simulink model "sldemo_tank"  (R2019b)
settings: Solver=ode1  StartTime=0.0  StopTime=170  FixedStep=.5  RelTol=1e-3  AbsTol=1e-6
PreLoadFcn:
  | sldemo_tankgui
StartFcn:
  | sldemo_tankgui start
StopFcn:
  | sldemo_tankgui stop
undefined symbols (not defined in the file): area, hilim, inflow, lolim, outflow, sigbuilder_block
CloseFcn:
  | sldemo_tankgui done
Description:
  | Tank Fill and Empty with Animation
  | 
  | This example shows how to model the dynamics of liquid in a tank. The
  | associated animation provides a graphical display of the tank as it empties and
  | refills, based on user-defined tank parameters. The tank empties at the start
  | of the simulation and again part way through the simulation. When the simulation
  | is stopped, a plot is generated showing the liquid height and the states of the
  | two valves.
settings Model: ExtModeTrigMode=oneshot  ExtModeArmWhenConnect=off  ExtModeAutoUpdateStatusClock=off  Creator=The MathWorks, Inc.  LastModifiedBy=The MathWorks, Inc.
settings SolverCC: AutoScaleAbsTol=off
settings DataIOCC: SaveFormat=Array  ReturnWorkspaceOutputs=off  SignalLoggingName=sigsOut
settings OptimizationCC: InitFltsAndDblsToZero=on  LifeSpan=inf  BufferReusableBoundary=off
settings DebuggingCC: SaveWithParameterizedLinksMsg=none  UnderspecifiedInitializationDetection=Classic  MergeDetectMultiDrivingBlocksExec=none  SignalResolutionControl=TryResolveAllWithWarning  MultiTaskDSMMsg=warning  MultiTaskCondExecSysMsg=none  IntegerOverflowMsg=none  FcnCallInpInsideContextMsg=warning  BusObjectLabelMismatch=none  StateNameClashWarn=warning  SFUnexpectedBacktrackingDiag=warning  SFNoUnconditionalDefaultTransitionDiag=warning  SFExecutionAtInitializationDiag=none  IntegerSaturationMsg=none  ArithmeticOperatorsInVariantConditions=warning
settings HardwareCC: ProdBitPerPointer=32  ProdBitPerSizeT=32  ProdBitPerPtrDiffT=32  ProdLargestAtomicFloat=None  ProdIntDivRoundTo=Undefined  ProdEndianess=Unspecified  ProdWordSize=32  ProdHWDeviceType=32-bit Generic  TargetUnknown=on
settings ModelReferenceCC: PropagateSignalLabelsOutOfModel=off
settings SFSimCC: SimUseLocalCustomCode=off  CustomCodeUndefinedFunction=UseInterfaceOnly
settings RTWCC: Description=Generic Real-Time Target  RTWUseLocalCustomCode=off
settings CodeAppCC: StateflowObjectComments=on
settings GRTTargetCC: TargetFcnLib=ansi_tfl_tmw.mat  TargetLangStandard=C89/C90 (ANSI)  GeneratePreprocessorConditionals=Disable all  CombineOutputUpdateFcns=off  GRTInterface=on
settings ConfigComp: CovMetricSettings=dw  CovHtmlReporting=on  CovSaveCumulativeToWorkspaceVar=on  CovSaveSingleToWorkspaceVar=on  CovExternalEMLEnable=off

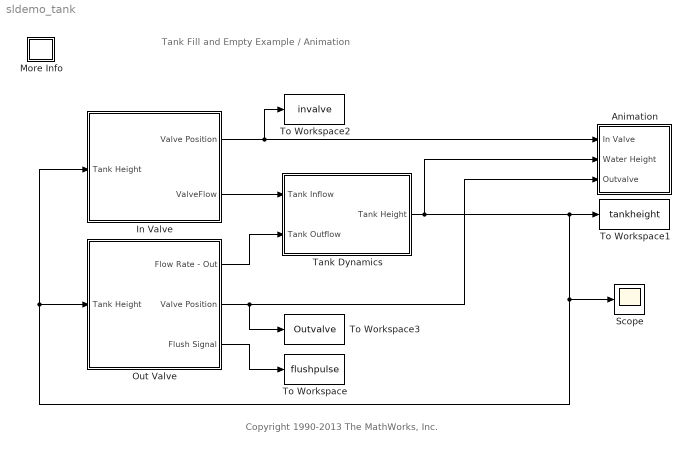
== system sldemo_tank ==
  note: Tank Fill and Empty Example / Animation
  note: Copyright 1990-2013 The MathWorks, Inc.
  Animation : Subsystem
      mask Display: disp('Animation\nControl')
  In Valve : Subsystem  mask{hilim=hilim, inflow=inflow}
      mask prompts: hilim "Shut Off Height"; inflow "Flow Rate"
  More Info : Subsystem
      settings: OpenFcn=showExample('simulink_general/sldemo_tankExample')
      mask Display: disp('?')
  Out Valve : Subsystem
  Scope : Scope
  Tank Dynamics : Subsystem
  To Workspace : ToWorkspace  VariableName=flushpulse  SampleTime=-1
  To Workspace1 : ToWorkspace  VariableName=tankheight  SampleTime=-1
  To Workspace2 : ToWorkspace  VariableName=invalve  SampleTime=-1
  To Workspace3 : ToWorkspace  VariableName=Outvalve  SampleTime=-1
  wires:
  Out Valve/2(Valve Position) -> Animation/3(Outvalve), To Workspace3/1
  In Valve/1(Valve Position) -> Animation/1(In Valve), To Workspace2/1
  Tank Dynamics/1(Tank Height) -> Animation/2(Water Height), Scope/1, In Valve/1(Tank Height), Out Valve/1(Tank Height), To Workspace1/1
  In Valve/2(ValveFlow) -> Tank Dynamics/1(Tank Inflow)
  Out Valve/1(Flow Rate - Out) -> Tank Dynamics/2(Tank Outflow)
  Out Valve/3(Flush Signal) -> To Workspace/1

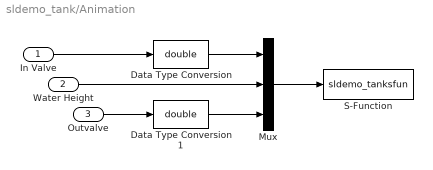
== system sldemo_tank/Animation ==
  In Valve : Inport
  Water Height : Inport  Port=2
  Outvalve : Inport  Port=3
  Data Type Conversion : DataTypeConversion  OutDataTypeStr=double  SaturateOnIntegerOverflow=on  RndMeth=Zero
  Data Type Conversion1 : DataTypeConversion  OutDataTypeStr=double  SaturateOnIntegerOverflow=on  RndMeth=Zero
  Mux : Mux  Inputs=3
  S-Function : S-Function  FunctionName=sldemo_tanksfun  Parameters=inflow,outflow,lolim,hilim,area  SFunctionDeploymentMode=off  EnableBusSupport=off
  wires:
  Outvalve/1 -> Data Type Conversion1/1
  Water Height/1 -> Mux/2
  Mux/1 -> S-Function/1
  In Valve/1 -> Data Type Conversion/1
  Data Type Conversion1/1 -> Mux/3
  Data Type Conversion/1 -> Mux/1

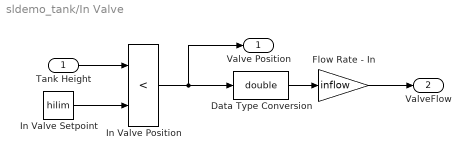
== system sldemo_tank/In Valve ==
  Tank Height : Inport
  Data Type Conversion : DataTypeConversion  OutDataTypeStr=double  SaturateOnIntegerOverflow=on  RndMeth=Zero
  Flow Rate - In : Gain  Gain=inflow  OutDataTypeStr=Inherit: Inherit via back propagation  SaturateOnIntegerOverflow=on  ParamDataTypeStr=Inherit: Same as input
  In Valve Position : RelationalOperator  Operator=<  RndMeth=Nearest  InputSameDT=on
  In Valve Setpoint : Constant  Value=hilim
  Valve Position : Outport  InitialOutput=0  VectorParamsAs1DForOutWhenUnconnected=off
  ValveFlow : Outport  Port=2  InitialOutput=0  VectorParamsAs1DForOutWhenUnconnected=off
  wires:
  Flow Rate - In/1 -> ValveFlow/1
  In Valve Position/1 -> Valve Position/1, Data Type Conversion/1
  Tank Height/1 -> In Valve Position/1
  In Valve Setpoint/1 -> In Valve Position/2
  Data Type Conversion/1 -> Flow Rate - In/1

== system sldemo_tank/More Info ==

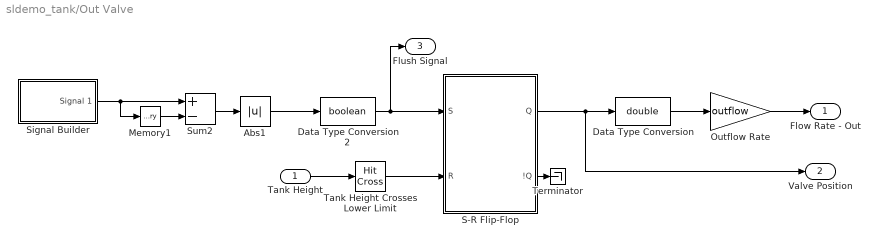
== system sldemo_tank/Out Valve ==
  Tank Height : Inport
  Abs1 : Abs  SaturateOnIntegerOverflow=on
  Data Type Conversion2 : DataTypeConversion  OutDataTypeStr=boolean  SaturateOnIntegerOverflow=on  RndMeth=Zero
  Data Type Conversion : DataTypeConversion  OutDataTypeStr=double  SaturateOnIntegerOverflow=on  RndMeth=Zero
  Memory1 : Memory
  Outflow Rate : Gain  Gain=outflow  SaturateOnIntegerOverflow=on  OutDataTypeStr=Inherit: Same as input  ParamDataTypeStr=Inherit: Same as input
  S-R Flip-Flop : Subsystem  mask(S-R Flip-Flop){}
  Signal Builder : Subsystem  Tag=STV Subsys  LoadFcn=sigbuilder_block('load');  StartFcn=sigbuilder_block('start');  StopFcn=sigbuilder_block('stop');  ClipboardFcn=sigbuilder_block('clipboard');  mask(Sigbuilder block){tuvar=[0:10]}
      mask help: Sigbuilder GUI
      mask init:
      | if ~strcmp(get_param(bdroot(gcb),'SimulationStatus'),'stopped') tuvar = sigbuilder_block('maskInit'); end
      settings: CopyFcn=sigbuilder_block('copy');  DeleteFcn=sigbuilder_block('delete');  ModelCloseFcn=sigbuilder_block('modelClose');  PreSaveFcn=sigbuilder_block('preSave');  PauseFcn=sigbuilder_block('pause')  ContinueFcn=sigbuilder_block('continue')  NameChangeFcn=sigbuilder_block('namechange');  OpenFcn=sigbuilder_block('open',[87.75 166.5 618.75 375 ]);  CloseFcn=sigbuilder_block('close');
      mask Display: plot(0, 0, 100, 100,[2, 2, 32, 32, 2], [68, 8, 8, 68, 68],[32, 2], [38, 38], [32, 19, 2],[53, 60, 44], [32, 17, 17, 2],[16, 16, 31, 31]);txt = getActiveGroup(gcbh);text(2, 100, txt,'verticalAlignment', 'top');
  Sum2 : Sum  Inputs=+-  SaturateOnIntegerOverflow=on  InputSameDT=on  OutDataTypeStr=Inherit: Same as first input
  Tank Height Crosses Lower Limit : HitCross  HitCrossingOffset=lolim  HitCrossingDirection=falling
  Terminator : Terminator
  Flow Rate - Out : Outport  InitialOutput=0  VectorParamsAs1DForOutWhenUnconnected=off
  Valve Position : Outport  Port=2  InitialOutput=0  VectorParamsAs1DForOutWhenUnconnected=off
  Flush Signal : Outport  Port=3  InitialOutput=0  VectorParamsAs1DForOutWhenUnconnected=off
  wires:
  Tank Height/1 -> Tank Height Crosses Lower Limit/1
  Tank Height Crosses Lower Limit/1 -> S-R Flip-Flop/2(R)
  S-R Flip-Flop/1(Q) -> Valve Position/1, Data Type Conversion/1
  S-R Flip-Flop/2(!Q) -> Terminator/1
  Outflow Rate/1 -> Flow Rate - Out/1
  Data Type Conversion/1 -> Outflow Rate/1
  Data Type Conversion2/1 -> S-R Flip-Flop/1(S), Flush Signal/1
  Signal Builder/1(Signal 1) -> Sum2/1, Memory1/1
  Sum2/1 -> Abs1/1
  Memory1/1 -> Sum2/2
  Abs1/1 -> Data Type Conversion2/1

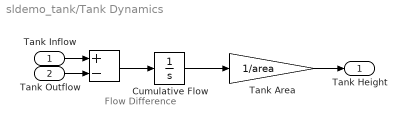
== system sldemo_tank/Tank Dynamics ==
  note: Flow
      | Difference
  Tank Inflow : Inport
  Tank Outflow : Inport  Port=2
  " " : Sum  Inputs=+-  SaturateOnIntegerOverflow=on  InputSameDT=on  OutDataTypeStr=Inherit: Same as first input
  Cumulative Flow : Integrator  InitialCondition=(hilim+lolim)/2*area
  Tank Area : Gain  Gain=1/area  SaturateOnIntegerOverflow=on  OutDataTypeStr=Inherit: Same as input  ParamDataTypeStr=Inherit: Same as input
  Tank Height : Outport  InitialOutput=0  VectorParamsAs1DForOutWhenUnconnected=off
  wires:
  Tank Outflow/1 -> " "/2
  Tank Inflow/1 -> " "/1
  " "/1 -> Cumulative Flow/1
  Cumulative Flow/1 -> Tank Area/1
  Tank Area/1 -> Tank Height/1

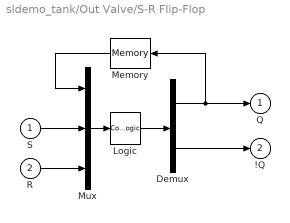
== system sldemo_tank/Out Valve/S-R Flip-Flop ==
  S : Inport
  R : Inport  Port=2
  Demux : Demux  Outputs=2
  Logic : CombinatorialLogic  TruthTable=[0 1;0 1;1 0;0 1;1 0;0 1;1 0;1 0]
  Memory : Memory  InheritSampleTime=on
  Mux : Mux  Inputs=3
  Q : Outport  InitialOutput=0  VectorParamsAs1DForOutWhenUnconnected=off
  !Q : Outport  Port=2  InitialOutput=1  VectorParamsAs1DForOutWhenUnconnected=off
  wires:
  R/1 -> Mux/3
  S/1 -> Mux/2
  Memory/1 -> Mux/1
  Demux/1 -> Memory/1, Q/1
  Demux/2 -> !Q/1
  Logic/1 -> Demux/1
  Mux/1 -> Logic/1

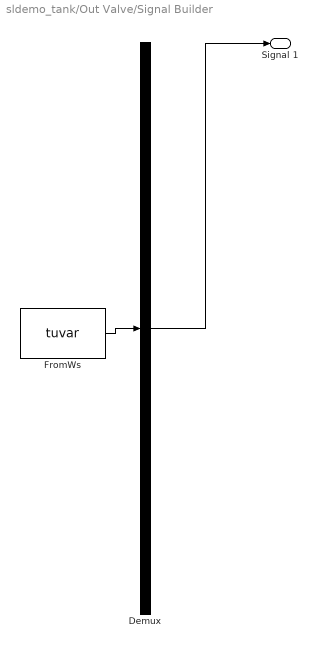
== system sldemo_tank/Out Valve/Signal Builder ==
  Demux : Demux  Tag=STV Demux  Outputs=1
  FromWs : FromWorkspace  Tag=STV FromWs  VariableName=tuvar  SampleTime=0
      SigBuilderData=|
      | dataSet.timeRange = [0 150]
      | dataSet.name = 'Group 1'
      | sbobj.Groups.Name = 'Group 1'
      | sbobj.Groups.Signals.Name = 'Signal 1'
      | sbobj.Groups.Signals.XData = [0 50 50 150]
      | sbobj.Groups.Signals.YData = [0 0 1 1]
      | sbobj.Groups.TimeRange = [0 150]
  Signal 1 : Outport  Tag=STV Outport  VectorParamsAs1DForOutWhenUnconnected=off
  wires:
  FromWs/1 -> Demux/1
  Demux/1 -> Signal 1/1
